simulink model "OW1_rev1"  (R2025b)
settings: Solver=ode4  StartTime=0  StopTime=120  FixedStep=0.005  MaxStep=0.005  RelTol=1e-3
values from neighbouring files (symbols this model uses):
  HP_unstretched_length = 0.4064*2    (= 0.8128)    [wecSimInputFile.m]
undefined symbols (not defined in the file or in its folder): body, cable, constraint, geometry, hydroData, pto
libraries: hose_pump_unit_v4 x4, nesl_utility x2, WECSim_Lib_Constraints x2, WECSim_Lib_Cables x1, WECSim_Lib_Frames x1, fl_lib x1, WECSim_Lib_Body_Elements x1, sm_lib x1, WECSim_Lib_PTOs x1
settings Model: Creator=cmmcguir  LastModifiedBy=cmmcguir
settings SolverCC: ZeroCrossControl=DisableAll  AutoInsertRateTranBlk=on
settings DataIOCC: ReturnWorkspaceOutputs=off
settings OptimizationCC: SimCompilerOptimization=on
settings RTWCC: GPUComputeCapability=3.5
settings SimscapeCC: SimscapeLogType=all  SimscapeLogLimitData=off

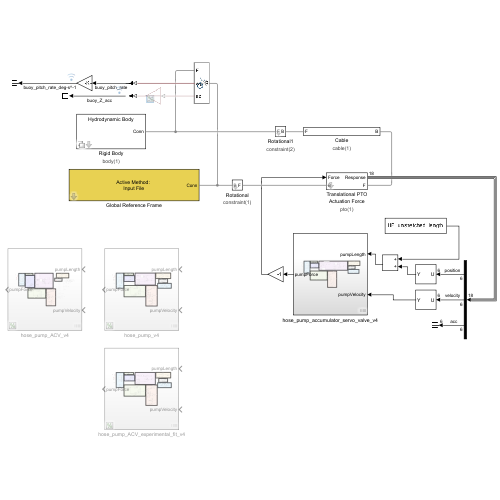
[thumbnail: Simulink's stored preview of the top-level diagram]
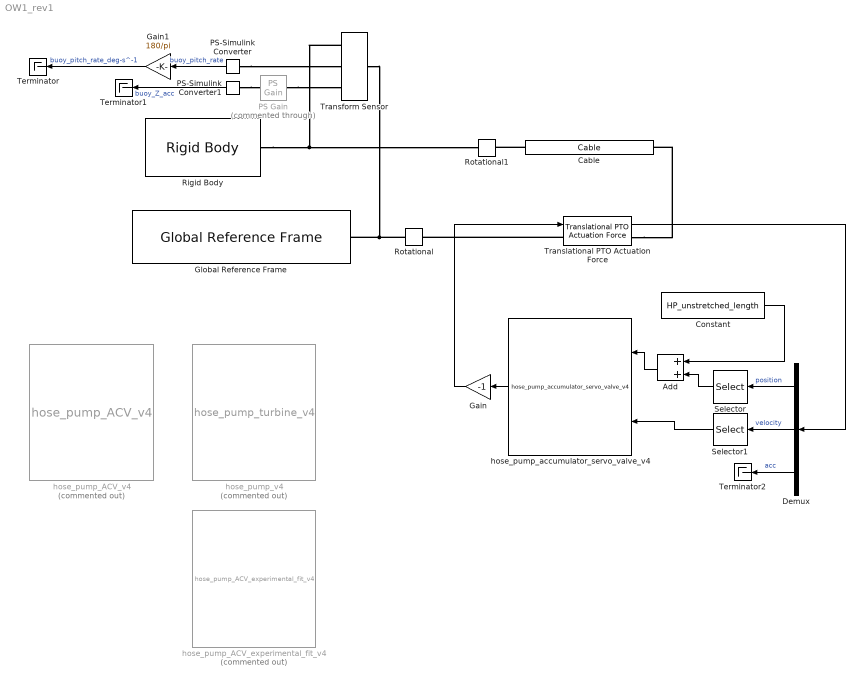
== system OW1_rev1 ==
  Add : Sum
  Cable : WECSim_Lib_Cables/Cable  VariantControl=sv_Cable3DOF  cable=cable(1)  baseConnectionName=constraint(1)  followerConnectionName=constraint(2)  stiffness=0  damping=0  length=0  preTension=0  diplacement=0 0 0  axis=0 1 0  angle=0  y=0 1 0  z=0 0 1
      settings: AttributesFormatString=%<cable>
  Constant : Constant  Value=HP_unstretched_length
  Demux : Demux  Outputs=3
  Gain : Gain  Gain=-1
  Gain1 : Gain  Gain=180/pi
  Global Reference Frame : WECSim_Lib_Frames/Global Reference Frame  waves=waves  simu=simu  InputMethod=Input File  InputFile=wecSimInputFile.m  mode=normal  explorer=off  solver=ode4  startTime=0  rampTime=100  endTime=400  dt=0.1  cicEndTime=60  stateSpace=0  WaveClass=regular  height=2.5  period=8  elevationFile=NOT DEFINED  spectrumFile=NOT DEFINED  direction=0  spread=1  spectrumType=NOT DEFINED  phaseSeed=0  option=EqualEnergy
  PS Gain : fl_lib/Physical Signals/Functions/PS Gain  Commented=through  gain=-1
  PS-Simulink Converter : nesl_utility/PS-Simulink Converter  PhysicalDomain=network_engine_domain  SubClassName=ps_output  LeftPortType=input  RightPortType=output  PseudoPeriodic=off  Frequencies=[]  VectorFormat=inherit  Unit=inherit  AffineConversion=off
  PS-Simulink Converter1 : nesl_utility/PS-Simulink Converter  PhysicalDomain=network_engine_domain  SubClassName=ps_output  LeftPortType=input  RightPortType=output  PseudoPeriodic=off  Frequencies=[]  VectorFormat=inherit  Unit=inherit  AffineConversion=off
  Rigid Body : WECSim_Lib_Body_Elements/Rigid Body  body=body(1)  h5File=hydroData/*.h5  geometryFile=geometry/*.stl  mass=0  inertia=0 0 0  inertiaProducts=0 0 0  nonHydro=0  nonlinearHydro=0  centerGravity=0 0 0  centerBuoyancy=0 0 0  dof=6  volume=0  QTFs=0  displacement=0 0 0  axis=0 1 0  angle=0  option=0  cd=0 0 0  ca=0 0 0  area=0 0 0  VME=0  rgME=0 0 0  z=0 0 1
  Rotational : WECSim_Lib_Constraints/Rotational  constraint=constraint(1)  loc="0  0  0"  displacement=0 0 0  y=0 1 0  z=0 0 1  upperLimitSpecify=off  upperLimitBound=0  upperLimitTransitionRegionWidth=0  upperLimitStiffness=0  upperLimitDamping=0  lowerLimitSpecify=off  lowerLimitBound=0  lowerLimitTransitionRegionWidth=0  lowerLimitStiffness=0  lowerLimitDamping=0
      settings: AttributesFormatString=%<constraint>
  Rotational1 : WECSim_Lib_Constraints/Rotational  constraint=constraint(2)  loc="0  0  0"  displacement=0 0 0  y=0 1 0  z=0 0 1  upperLimitSpecify=off  upperLimitBound=0  upperLimitTransitionRegionWidth=0  upperLimitStiffness=0  upperLimitDamping=0  lowerLimitSpecify=off  lowerLimitBound=0  lowerLimitTransitionRegionWidth=0  lowerLimitStiffness=0  lowerLimitDamping=0
      settings: AttributesFormatString=%<constraint>
  Selector : Selector  InputPortWidth=6  IndexOptions=Index vector (dialog)  Indices=3  OutputSizes=1
  Selector1 : Selector  InputPortWidth=6  IndexOptions=Index vector (dialog)  Indices=3  OutputSizes=1
  Terminator : Terminator
  Terminator1 : Terminator
  Terminator2 : Terminator
  Transform Sensor : sm_lib/Frames and Transforms/Transform Sensor  MeasurementFrame=World  RotationSequence=XYX  SenseAngle=off  SenseAxis=off  SenseQ=off  SenseR=off  SenseRotationSequence=off  SenseOmegaX=off  SenseOmegaY=on  SenseOmegaZ=off  SenseOmega=off  SenseQDot=off  SenseRDot=off  SenseRotationSequenceDot=off  SenseAlphaX=off  SenseAlphaY=off  SenseAlphaZ=off  SenseAlpha=off  SenseQDDot=off  SenseRDDot=off  SenseX=off  SenseY=off  SenseZ=off  SenseXYZ=off  SenseRad=off  SenseAzim=off  SenseDist=off  SenseInc=off  SenseXDot=off  SenseYDot=off  SenseZDot=off  SenseXYZDot=off  SenseRadDot=off  SenseAzimDot=off  SenseDistDot=off  SenseIncDot=off  SenseXDDot=off  SenseYDDot=off  SenseZDDot=on  SenseXYZDDot=off  SenseRadDDot=off  SenseAzimDDot=off  SenseDistDDot=off  SenseIncDDot=off
  Translational PTO Actuation Force : WECSim_Lib_PTOs/Translational PTO Actuation Force  pto=pto(1)  loc="0  0  0"  stiffness=0  damping=0  equilibriumPosition=0  pretension=0  displacement=0 0 0  y=0 1 0  z=0 0 1  upperLimitSpecify=off  upperLimitBound=0  upperLimitTransitionRegionWidth=0  upperLimitStiffness=0  upperLimitDamping=0  lowerLimitSpecify=off  lowerLimitBound=0  lowerLimitTransitionRegionWidth=0  lowerLimitStiffness=0  lowerLimitDamping=0
      settings: AttributesFormatString=%<pto>
  hose_pump_ACV_experimental_fit_v4 : hose_pump_unit_v4/hose_pump_ACV_experimental_fit_v4  Commented=on  SystemSampleTime=-1  VariantActivationTime=update diagram  EmptyChoice=off  PassThrough=off  PassThroughVariantControl=(default)  EmptyChoiceVariantControl=(default)  AllowFlexibleInterface=on  Latency=0  AutoFrameSizeCalculation=off
  hose_pump_ACV_v4 : hose_pump_unit_v4/hose_pump_ACV_v4  Commented=on  SystemSampleTime=-1  VariantActivationTime=update diagram  EmptyChoice=off  PassThrough=off  PassThroughVariantControl=(default)  EmptyChoiceVariantControl=(default)  AllowFlexibleInterface=on  Latency=0  AutoFrameSizeCalculation=off
  hose_pump_accumulator_servo_valve_v4 : hose_pump_unit_v4/hose_pump_accumulator_servo_valve_v4  SystemSampleTime=-1  VariantActivationTime=update diagram  EmptyChoice=off  PassThrough=off  PassThroughVariantControl=(default)  EmptyChoiceVariantControl=(default)  AllowFlexibleInterface=on  Latency=0  AutoFrameSizeCalculation=off
  hose_pump_v4 : hose_pump_unit_v4/hose_pump_turbine_v4  Commented=on  SystemSampleTime=-1  VariantActivationTime=update diagram  EmptyChoice=off  PassThrough=off  PassThroughVariantControl=(default)  EmptyChoiceVariantControl=(default)  AllowFlexibleInterface=on  Latency=0  AutoFrameSizeCalculation=off
  wires:
  Demux/1 -> Selector/1  "position"
  Selector/1 -> Add/2
  Demux/2 -> Selector1/1  "velocity"
  Demux/3 -> Terminator2/1  "acc"
  Translational PTO Actuation Force/1 -> Demux/1
  hose_pump_accumulator_servo_valve_v4/1 -> Gain/1
  Add/1 -> hose_pump_accumulator_servo_valve_v4/1
  Constant/1 -> Add/1
  Gain/1 -> Translational PTO Actuation Force/1
  Selector1/1 -> hose_pump_accumulator_servo_valve_v4/2
  PS-Simulink Converter/1 -> Gain1/1  "buoy_pitch_rate"
  Gain1/1 -> Terminator/1  "buoy_pitch_rate_deg-s^-1"
  PS-Simulink Converter1/1 -> Terminator1/1  "buoy_Z_acc"
  connections:
  Cable/RConn1 -- Rotational1/LConn1
  Rotational/LConn1 -- Transform Sensor/LConn1 -- Global Reference Frame/RConn1
  Translational PTO Actuation Force/LConn1 -- Rotational/RConn1
  Translational PTO Actuation Force/RConn1 -- Cable/LConn1
  Rigid Body/RConn1 -- Transform Sensor/RConn1 -- Rotational1/RConn1
  PS-Simulink Converter/LConn1 -- Transform Sensor/RConn2
  PS-Simulink Converter1/LConn1 -- PS Gain/RConn1
  PS Gain/LConn1 -- Transform Sensor/RConn3
